simulink model "PSMPraga"  (R2021b)
settings: Solver=FixedStepDiscrete  StartTime=0.0  StopTime=8  RelTol=1e-3
PreLoadFcn:
  | Ts_Power=1e-6;
  | Ts_Control=100e-6;
undefined symbols (not defined in the file or in its folder): D1, Delta, DiscIntNeverNeededParam, sigbuilder_block
libraries: spsSeriesRLCBranchLib x10, spsVoltageMeasurementLib x10, slpidlib x8, spsPowerPositiveSequenceLib x8, spsCurrentMeasurementLib x8, spsThreePhaseVIMeasurementLib x6, eePowerMeasurement x6, spsabctodq0Lib x4, spsMeanLib x3, spsThreePhaseTransformerTwoWindingsLib x3, spsThreePhaseParallelRLCLoadLib x2, spsParallelRLCLoadLib x2
(part 1 of 3)
Description:
  | Copyright 2008-2019 The MathWorks, Inc.
settings Model: SimulationMode=accelerator  Creator=MathWorks  LastModifiedBy=user
settings SolverCC: AlgebraicLoopSolver=TrustRegion
settings DataIOCC: LimitDataPoints=on  SaveFormat=Array  SignalLoggingSaveFormat=ModelDataLogs  SignalLogging=off  DSMLogging=off  ReturnWorkspaceOutputs=off
settings OptimizationCC: ExpressionDepthLimit=2147483647  LifeSpan=inf
settings DebuggingCC: UnderspecifiedInitializationDetection=Classic  MergeDetectMultiDrivingBlocksExec=none  SolverPrmCheckMsg=warning  FcnCallInpInsideContextMsg=warning  StateNameClashWarn=warning  SFUnexpectedBacktrackingDiag=warning  SFNoUnconditionalDefaultTransitionDiag=warning  SFExecutionAtInitializationDiag=none  SFMachineParentedDataDiag=warning  ArithmeticOperatorsInVariantConditions=warning
settings HardwareCC: ProdBitPerPointer=32  ProdBitPerSizeT=32  ProdBitPerPtrDiffT=32  ProdLargestAtomicFloat=None  ProdIntDivRoundTo=Undefined  ProdEndianess=Unspecified  ProdWordSize=32  ProdHWDeviceType=32-bit Generic
settings ModelReferenceCC: PropagateSignalLabelsOutOfModel=off
settings SFSimCC: SimUseLocalCustomCode=off  CustomCodeUndefinedFunction=UseInterfaceOnly
settings RTWCC: RTWUseLocalCustomCode=off
settings CodeAppCC: StateflowObjectComments=on
settings GRTTargetCC: TargetLangStandard=C89/C90 (ANSI)  CombineOutputUpdateFcns=off  GRTInterface=on
settings ConfigComp: CovMetricSettings=dw  CovSaveCumulativeToWorkspaceVar=on  CovSaveSingleToWorkspaceVar=on  CovExternalEMLEnable=off  CovSFcnEnable=off
settings SimscapeCC: SimscapeNormalizeSystem=off

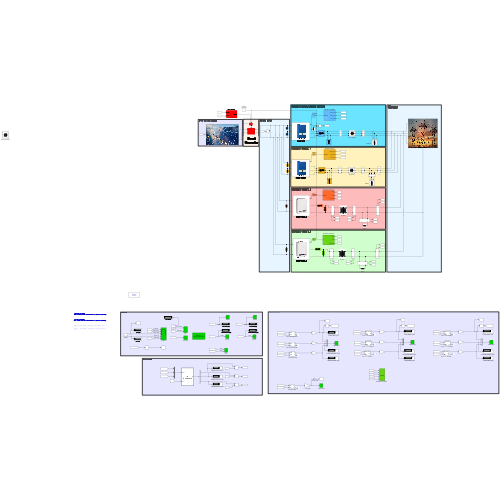
[thumbnail: Simulink's stored preview of the top-level diagram]
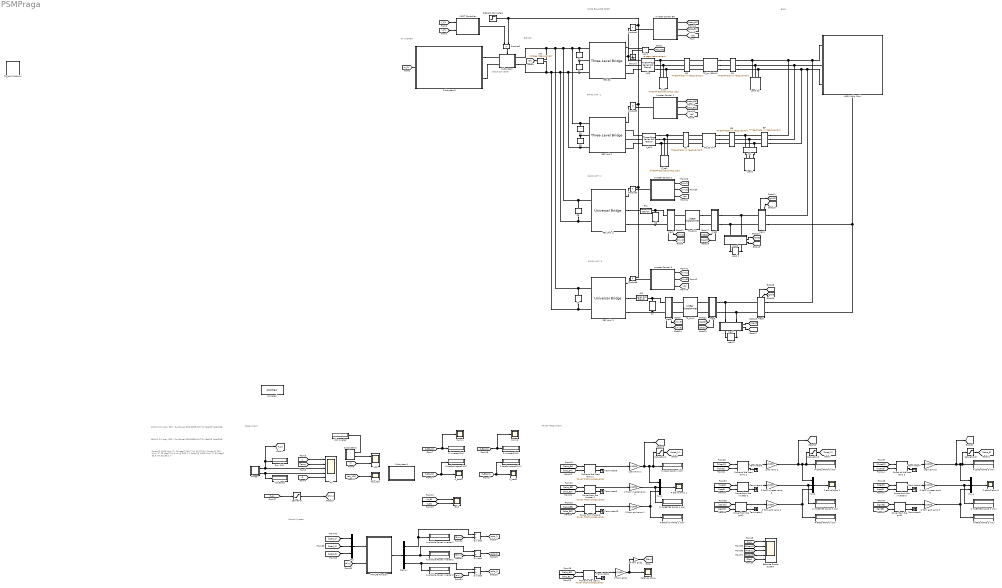
== system PSMPraga ==
  note: GRID
  note: RAMO UNIT. 3
  note: RAMO UNIT. 2
  note: RAMO UNIT. 1
  note: RAMO BALANCE NODE
  note: BUS DC
  note: PV SYSTEM
  note: Power Measurment
  note: Measurment
  note: Control System
  note: Boost Converter
  note: Pmpp @ 1000 W/m^2, 25 deg= 100.7 kW @ 273.5 V
      | Pmpp @  250 W/m^2, 25 deg= 24.4  kW @ 265.1 V
      | Pmpp @ 1000 W/m^2, 50 deg= 92.9  kW @ 250.2 V
  note: 100-kW  PV Array
      | 330 * SunPower SPR-305E-WHT-D  (Nser=5 Npar=66)
  note: 100-kW  PV Array
      | 330 * SunPower SPR-305E-WHT-D  (Nser=5 Npar=66)
  " Load SC" : spsThreePhaseParallelRLCLoadLib/Three-Phase Parallel RLC Load  LConnTagsString=A|B|C  Configuration=Y (grounded)  NominalVoltage=400  Vabc=[1e3 1e3 1e3]  Vabcp=[1e3 1e3 1e3]  NominalFrequency=50  UnbalancedPower=off  ActivePower=0.1  InductivePower=0  CapacitivePower=0  Pabc=[10e3 9e3 11e3]  QLabc=[100 90 110]  QCabc=[100 90 110]  Pabcp=[10e3 9e3 11e3]  QLabcp=[100 90 110]  QCabcp=[100 90 110]  Measurements=None  LoadType=constant Z
  " Load1" : spsThreePhaseParallelRLCLoadLib/Three-Phase Parallel RLC Load  LConnTagsString=A|B|C  Configuration=Y (grounded)  NominalVoltage=400  Vabc=[1e3 1e3 1e3]  Vabcp=[1e3 1e3 1e3]  NominalFrequency=50  UnbalancedPower=off  ActivePower=10000  InductivePower=0  CapacitivePower=0  Pabc=[10e3 9e3 11e3]  QLabc=[100 90 110]  QCabc=[100 90 110]  Pabcp=[10e3 9e3 11e3]  QLabcp=[100 90 110]  QCabcp=[100 90 110]  Measurements=None  LoadType=constant Z
  " Load 3" : spsParallelRLCLoadLib/Parallel RLC Load  LConnTagsString=a  RConnTagsString=__new0  NominalVoltage=230  NominalFrequency=50  ActivePower=3000  InductivePower=0  CapacitivePower=0  Setx0=off  InitialVoltage=0  SetiL0=off  InitialCurrent=0  Measurements=None  LoadType=constant Z
      settings: AttributesFormatString=\n  SourceProductBaseCode=PS
  600V Utlity Grid : Subsystem
      settings: PortSchema="{\"entries\":[{\"content\":{\"sides\":[{\"content\":{\"connectorIds\":[\"LConn1\",\"LConn2\",\"LConn3\"]},\"type\":\"ConnectorPlacement.EquallySpacedRectSide\",\"uuid\":\"36023811-46b7-429e-a8ab-d56566142e79\"},{\"content\":{\"connectorIds\":[],\"side\":\"RIGHT\"},\"type\":\"ConnectorPlacement.EquallySpacedRectSide\",\"uuid\":\"9af551aa-fa19-4e35-bdf3-eccb9cb0d58d\"},{\"content\":{\"connectorIds\":[],\"side\":\"TOP\"},\"type\":\"ConnectorPlacement.EquallySpacedRectSide\",\"uuid\":\"a2a5be34-f490-4bba-9aee-93a63d2f5fd5\"},{\"content\":{\"connectorIds\":[\"RConn1\"],\"side\":\"BOTTOM\"},\"type\":\"ConnectorPlacement.EquallySpacedRectSide\",\"uuid\":\"ebfc3acd-3bb4-47e0-af2a-a9fa1738ee4a\"}]},\"type\":\"ConnectorPlacement.EquallySpacedConnector\",\"uuid\":\"d54a4b0f-3adc-4ffb-80dc-ac1d592a2d32\"}],\"packageUris\":[\"http://schema.mathworks.com/mf0/Connector/R2020b\"],\"version\":\"1.0\"}"
      mask Display: image('$imagefile'); % Use "Edit Image" on toolstrip to change.
  Available Power Inverter 1 : Display
  Available Power Inverter 2 : Display
  Available Power Inverter 3 : Display
  B0 : spsThreePhaseVIMeasurementLib/Three-Phase V-I Measurement  VoltageMeasurement=phase-to-ground  SetLabelV=on  LabelV=Vabc_B0  Vpu=off  VpuLL=off  CurrentMeasurement=yes  SetLabelI=on  LabelI=Iabc_B0  Ipu=off  Pbase=100e6  Vbase=500e3  OutputType=Magnitude  PhasorSimulation=off  PSBequivalent=0
  B1 : spsThreePhaseVIMeasurementLib/Three-Phase V-I Measurement  VoltageMeasurement=phase-to-ground  SetLabelV=on  LabelV=Vabc_B1  Vpu=off  VpuLL=off  CurrentMeasurement=yes  SetLabelI=on  LabelI=Iabc_B1  Ipu=off  Pbase=100e6  Vbase=500e3  OutputType=Magnitude  PhasorSimulation=off  PSBequivalent=0
  B2 : spsThreePhaseVIMeasurementLib/Three-Phase V-I Measurement  VoltageMeasurement=phase-to-ground  SetLabelV=on  LabelV=Vabc_B2  Vpu=off  VpuLL=off  CurrentMeasurement=yes  SetLabelI=on  LabelI=Iabc_B2  Ipu=off  Pbase=100e6  Vbase=500e3  OutputType=Magnitude  PhasorSimulation=off  PSBequivalent=0
  B3 : spsThreePhaseVIMeasurementLib/Three-Phase V-I Measurement  VoltageMeasurement=phase-to-ground  SetLabelV=on  LabelV=Vabc_B3  Vpu=off  VpuLL=off  CurrentMeasurement=yes  SetLabelI=on  LabelI=Iabc_B3  Ipu=off  Pbase=100e6  Vbase=500e3  OutputType=Magnitude  PhasorSimulation=off  PSBequivalent=0
  B4 : spsThreePhaseVIMeasurementLib/Three-Phase V-I Measurement  VoltageMeasurement=phase-to-ground  SetLabelV=on  LabelV=Vabc_B4  Vpu=off  VpuLL=off  CurrentMeasurement=yes  SetLabelI=on  LabelI=Iabc_B4  Ipu=off  Pbase=100e6  Vbase=500e3  OutputType=Magnitude  PhasorSimulation=off  PSBequivalent=0
  B5 : spsThreePhaseVIMeasurementLib/Three-Phase V-I Measurement  VoltageMeasurement=phase-to-ground  SetLabelV=on  LabelV=Vabc_B5  Vpu=off  VpuLL=off  CurrentMeasurement=yes  SetLabelI=on  LabelI=Iabc_B5  Ipu=off  Pbase=100e6  Vbase=500e3  OutputType=Magnitude  PhasorSimulation=off  PSBequivalent=0
  Balance Power System : Scope  NumInputPorts=5
  C1 : spsSeriesRLCBranchLib/Series RLC Branch  LConnTagsString=__new0  RConnTagsString=__new0  BranchType=C  Resistance=1.0  Inductance=1.0  SetiL0=off  InitialCurrent=0  Capacitance=12000e-06  Setx0=off  InitialVoltage=0  Measurements=None
  C2 : spsSeriesRLCBranchLib/Series RLC Branch  LConnTagsString=__new0  RConnTagsString=__new0  BranchType=C  Resistance=1.0  Inductance=1.0  SetiL0=off  InitialCurrent=0  Capacitance=12000e-06  Setx0=off  InitialVoltage=0  Measurements=None
  C4 : spsSeriesRLCBranchLib/Series RLC Branch  LConnTagsString=__new0  RConnTagsString=__new0  BranchType=C  Resistance=1.0  Inductance=1.0  SetiL0=off  InitialCurrent=0  Capacitance=3000e-06  Setx0=off  InitialVoltage=0  Measurements=None
  C5 : spsSeriesRLCBranchLib/Series RLC Branch  LConnTagsString=__new0  RConnTagsString=__new0  BranchType=C  Resistance=1.0  Inductance=1.0  SetiL0=off  InitialCurrent=0  Capacitance=3000e-06  Setx0=off  InitialVoltage=0  Measurements=None
  C6 : spsSeriesRLCLoadLib/Series RLC Load  LConnTagsString=a  RConnTagsString=__new0  NominalVoltage=240  NominalFrequency=50  ActivePower=10e3/100  InductivePower=0  CapacitivePower=10e3  Setx0=off  InitialVoltage=0  SetiL0=off  InitialCurrent=0  Measurements=None  LoadType=constant Z
  C7 : spsSeriesRLCLoadLib/Series RLC Load  LConnTagsString=a  RConnTagsString=__new0  NominalVoltage=260  NominalFrequency=50  ActivePower=10e3/100  InductivePower=0  CapacitivePower=10e3  Setx0=off  InitialVoltage=0  SetiL0=off  InitialCurrent=0  Measurements=None  LoadType=constant Z
  C8 : spsSeriesRLCBranchLib/Series RLC Branch  LConnTagsString=__new0  RConnTagsString=__new0  BranchType=C  Resistance=1.0  Inductance=1.0  SetiL0=off  InitialCurrent=0  Capacitance=9000e-06  Setx0=off  InitialVoltage=0  Measurements=None
  C9 : spsSeriesRLCBranchLib/Series RLC Branch  LConnTagsString=__new0  RConnTagsString=__new0  BranchType=C  Resistance=1.0  Inductance=1.0  SetiL0=off  InitialCurrent=0  Capacitance=10000e-06  Setx0=off  InitialVoltage=0  Measurements=None
  C_ba : spsThreePhaseSeriesRLCLoadLib/Three-Phase Series RLC Load  LConnTagsString=A|B|C  Configuration=Y (grounded)  NominalVoltage=260  Vabc=[1e3 1e3 1e3]  Vabcp=[1e3 1e3 1e3]  NominalFrequency=50  UnbalancedPower=off  ActivePower=10e3/100  InductivePower=0  CapacitivePower=10e3  Pabc=[10e3 9e3 11e3]  QLabc=[100 90 110]  QCabc=[100 90 110]  Pabcp=[10e3 9e3 11e3]  QLabcp=[100 90 110]  QCabcp=[100 90 110]  Measurements=None  LoadType=constant Z
  C_ba1 : spsThreePhaseSeriesRLCLoadLib/Three-Phase Series RLC Load  LConnTagsString=A|B|C  Configuration=Y (grounded)  NominalVoltage=260  Vabc=[1e3 1e3 1e3]  Vabcp=[1e3 1e3 1e3]  NominalFrequency=50  UnbalancedPower=off  ActivePower=10e3/100  InductivePower=0  CapacitivePower=10e3  Pabc=[10e3 9e3 11e3]  QLabc=[100 90 110]  QCabc=[100 90 110]  Pabcp=[10e3 9e3 11e3]  QLabcp=[100 90 110]  QCabcp=[100 90 110]  Measurements=None  LoadType=constant Z
  Deblock Converters : Step  Time=0.05  SampleTime=0
  Demux : Demux  Outputs=3
  Divide3 : Product  Inputs=*/
  Divide4 : Product  Inputs=*/
  Divide5 : Product  Inputs=*/
  FEC BN : spsThreeLevelBridgeLib/Three-Level Bridge  Arms=3  SnubberResistance=1e6  SbubberCapacitance=inf  Device=IGBT / Diodes  Ron=0.2e-3  ForwardVoltages="[  0  0 ]"  Measurements=None  mask(Three-Level Bridge){}
      settings: AttributesFormatString=\n  SourceProductBaseCode=PS
      mask Display: image('C:\Users\user\Desktop\Matlab\Immagini\inverter trifase.jpg'); % Use "Edit Image" on toolstrip to change.
  FEC Unit. 2 : spsUniversalBridgeLib/Universal Bridge  Arms=2  SnubberResistance=1e6  SnubberCapacitance=inf  Device=IGBT / Diodes  Ron=0.2e-3  Lon=0  ForwardVoltages="[  0  0  ]"  ForwardVoltage=0  GTOparameters=[ 10e-6 , 20e-6 ]  IGBTparameters=[ 1e-6 , 2e-6 ]  Measurements=None  Measurements_2=None  converterType=Rectifier  mask(Universal Bridge){}
      mask Display: image('C:\Users\user\Desktop\Matlab\Immagini\inveter monofase.jpg'); % Use "Edit Image" on toolstrip to change.
  FEC Unit. 3 : spsUniversalBridgeLib/Universal Bridge  Arms=2  SnubberResistance=1e6  SnubberCapacitance=inf  Device=IGBT / Diodes  Ron=0.2e-3  Lon=0  ForwardVoltages="[  0  0  ]"  ForwardVoltage=0  GTOparameters=[ 10e-6 , 20e-6 ]  IGBTparameters=[ 1e-6 , 2e-6 ]  Measurements=None  Measurements_2=None  converterType=Rectifier  mask(Universal Bridge){}
      mask Display: image('C:\Users\user\Desktop\Matlab\Immagini\inveter monofase.jpg'); % Use "Edit Image" on toolstrip to change.
  FEC Unit.1 : spsThreeLevelBridgeLib/Three-Level Bridge  Arms=3  SnubberResistance=1e6  SbubberCapacitance=inf  Device=IGBT / Diodes  Ron=0.2e-3  ForwardVoltages="[0  0 ]"  Measurements=None  mask(Three-Level Bridge){}
      settings: AttributesFormatString=\n  SourceProductBaseCode=PS
      mask Display: image('C:\Users\user\Desktop\Matlab\Immagini\inverter trifase.jpg'); % Use "Edit Image" on toolstrip to change.
  Grid : Scope  NumInputPorts=2
  Ground : spsGroundLib/Ground  LConnTagsString=a
  Inverter Control 1 : Subsystem  mask(VSC Main Controller){nom=[10e3  50 ], Vnom=[400 260 ], Vnom_dc=500, RLxfo=[0.002  0.06], RLchoke=[0.0075 250e-6], K_VDCreg=[7 800], K_Ireg=[0.3 20], Ts=Ts_Control}
      mask prompts: nom "Nominal power and frequency [ Pnom(VA)  Fnom(Hz) ]:"; Vnom "Nominal primary and secondary voltages (Vrms LL) [ Vnom_prim   Vnom_sec ]:"; Vnom_dc "Nominal DC bus voltage (V):"; RLxfo "Total transformer leakage impedance (pu/Pnom) [ Rxfo  Lxf ]"; RLchoke "Choke impedance [ R(ohm) L(H) ]"; K_VDCreg "VDC regultator gains [ Kp  Ki ]:"; K_Ireg "Current regulator gains [ Kp  Ki ]:"; Ts "Sample time"
      mask init:
      | Pnom=nom(1);
      | Fnom=nom(2);
      | Vnom_prim=Vnom(1);
      | Vnom_sec=Vnom(2);
      | Zbase=(Vnom_sec^2/(Pnom*10));
      | Rtot_pu=RLxfo(1) + RLchoke(1)/Zbase;
      | Ltot_pu=RLxfo(2) + RLchoke(2)/(Zbase/(2*pi*Fnom));
      | Kp_VDCreg=K_VDCreg(1);
      | Ki_VDCreg=K_VDCreg(2);
      | Kp_Ireg=K_Ireg(1);
      | Ki_Ireg=K_Ireg(2);
      | Vdc_ref=Vnom_dc;
      | % Used to determine initial value of Boost Control (MPPT)
      | assignin('base','Vdc_ref_Inv',Vdc_ref);
  Inverter Control 2 : Subsystem  mask(Inverter Control){Pnom=6000, Fnom=50, Vnom_sec=260, Vnom_dc=500, Kp_VDCreg=7, Ki_VDCreg=800, Kp_Ireg=0.30, Ki_Ireg=20, RLxfo=[0.002  0.06], RLchoke=[2e-3  1.78e-3], Fc=1650, PWMmode12=Bipolar, Ts_Control=Ts_Control, Ts_PWMgenerator=Ts_Power}
      mask prompts: Pnom "Nominal Power (VA)"; Fnom "Frequency (Hz)"; Vnom_sec "Secondary voltage (Vrms LN)"; Vnom_dc "DC BUS voltage nominal (V)"; Kp_VDCreg "Proportional gain"; Ki_VDCreg "Integral gain"; Kp_Ireg "Proportional gain"; Ki_Ireg "Integral gain"; RLxfo "Total transformer leakage impedance (pu/Pnom) [ Rxfo  Lxf ]"; RLchoke "Choke impedance [ R(ohm) L(H) ]"; Fc "Carrier frequency (Hz)"; PWMmode12 "PWM method"; Ts_Control "Control systems"; Ts_PWMgenerator "PWM generator"
      mask help:
      | The main components of the Inverter Control are:
      | 1. PLL & Measurements
      | 2. Maximum Power Point Tracker System (MPPT) using a Perturb & Observe algorithm
      | 3. DC Voltage Regulator
      | 4. Current Regulator
      | 5. PWM Modulator
      mask init:
      | blockName=gcb;
      | Vdc_ref=Vnom_dc;
      | Zbase=Vnom_sec^2/(Pnom*3);
      | Rtot_pu=RLxfo(1) + RLchoke(1)/Zbase;
      | Ltot_pu=RLxfo(2) + RLchoke(2)/(Zbase/(2*pi*Fnom));
      | if PWMmode12==1
      |     set_param([blockName,'/','PWM_Generator'],'ModulatorType','Single-phase full-bridge (4 pulses)')
      | else
      |     set_param([blockName,'/','PWM_Generator'],'ModulatorType','Single-phase full-bridge - Bipolar modulation (4 pulses)')
      | end
      mask TypeOptions PWMmode12: Unipolar | Bipolar
      mask DialogControl Container4 Prompt: Nominal Values:
      mask DialogControl Container8 Prompt: Dc Voltage Regulator:
      mask DialogControl Container6 Prompt: Current Regulator:
      mask DialogControl Container9 Prompt: PWM Modulator:
      mask DialogControl SampleTimes Prompt: Sample Times:
  Inverter Control 3 : Subsystem  mask(Inverter Control){Pnom=3000, Fnom=50, Vnom_sec=260, Vnom_dc=500, Kp_VDCreg=7, Ki_VDCreg=800, Kp_Ireg=0.30, Ki_Ireg=20, RLxfo=[0.0002  0.000019], RLchoke=[2e-3  1.78e-3], Fc=1650, PWMmode12=Bipolar, Ts_Control=Ts_Control, Ts_PWMgenerator=Ts_Power}
      mask prompts: Pnom "Nominal Power (VA)"; Fnom "Frequency (Hz)"; Vnom_sec "Secondary voltage (Vrms LN)"; Vnom_dc "DC BUS voltage nominal (V)"; Kp_VDCreg "Proportional gain"; Ki_VDCreg "Integral gain"; Kp_Ireg "Proportional gain"; Ki_Ireg "Integral gain"; RLxfo "Total transformer leakage impedance (pu/Pnom) [ Rxfo  Lxf ]"; RLchoke "Choke impedance [ R(ohm) L(H) ]"; Fc "Carrier frequency (Hz)"; PWMmode12 "PWM method"; Ts_Control "Control systems"; Ts_PWMgenerator "PWM generator"
      mask help:
      | The main components of the Inverter Control are:
      | 1. PLL & Measurements
      | 2. Maximum Power Point Tracker System (MPPT) using a Perturb & Observe algorithm
      | 3. DC Voltage Regulator
      | 4. Current Regulator
      | 5. PWM Modulator
      mask init:
      | blockName=gcb;
      | Vdc_ref=Vnom_dc;
      | Zbase=Vnom_sec^2/Pnom;
      | Rtot_pu=RLxfo(1) + RLchoke(1)/Zbase;
      | Ltot_pu=RLxfo(2) + RLchoke(2)/(Zbase/(2*pi*Fnom));
      | if PWMmode12==1
      |     set_param([blockName,'/','PWM_Generator'],'ModulatorType','Single-phase full-bridge (4 pulses)')
      | else
      |     set_param([blockName,'/','PWM_Generator'],'ModulatorType','Single-phase full-bridge - Bipolar modulation (4 pulses)')
      | end
      mask TypeOptions PWMmode12: Unipolar | Bipolar
      mask DialogControl Container4 Prompt: Nominal Values:
      mask DialogControl Container8 Prompt: Dc Voltage Regulator:
      mask DialogControl Container6 Prompt: Current Regulator:
      mask DialogControl Container9 Prompt: PWM Modulator:
      mask DialogControl SampleTimes Prompt: Sample Times:
  Inverter Control BN : Subsystem  mask(VSC Main Controller){nom=[30e3  50 ], Vnom=[ 400 260 ], Vnom_dc=500, RLxfo=[0.002  0.06 ], RLchoke=[2e-3  250e-6  ], K_VDCreg=[7  800], K_Ireg=[0.3 20], Ts=Ts_Control}
      mask prompts: nom "Nominal power and frequency [ Pnom(VA)  Fnom(Hz) ]:"; Vnom "Nominal primary and secondary voltages (Vrms LL) [ Vnom_prim   Vnom_sec ]:"; Vnom_dc "Nominal DC bus voltage (V):"; RLxfo "Total transformer leakage impedance (pu/Pnom) [ Rxfo  Lxf ]"; RLchoke "Choke impedance [ R(ohm) L(H) ]"; K_VDCreg "VDC regultator gains [ Kp  Ki ]:"; K_Ireg "Current regulator gains [ Kp  Ki ]:"; Ts "Sample time"
      mask init:
      | Pnom=nom(1);
      | Fnom=nom(2);
      | Vnom_prim=Vnom(1);
      | Vnom_sec=Vnom(2);
      | Zbase=Vnom_sec^2/(Pnom*10/3);
      | Rtot_pu=RLxfo(1) + RLchoke(1)/Zbase;
      | Ltot_pu=RLxfo(2) + RLchoke(2)/(Zbase/(2*pi*Fnom));
      | Kp_VDCreg=K_VDCreg(1);
      | Ki_VDCreg=K_VDCreg(2);
      | Kp_Ireg=K_Ireg(1);
      | Ki_Ireg=K_Ireg(2);
      | Vdc_ref=Vnom_dc;
      | % Used to determine initial value of Boost Control (MPPT)
      | assignin('base','Vdc_ref_Inv',Vdc_ref);
  L_ba : spsThreePhaseSeriesRLCBranchLib/Three-Phase Series RLC Branch  LConnTagsString=A|B|C  RConnTagsString=A|B|C  BranchType=RL  Resistance=500e-6*377/50/2  Inductance=500e-6/2  Capacitance=inf  Measurements=None
  L_ba1 : spsThreePhaseSeriesRLCBranchLib/Three-Phase Series RLC Branch  LConnTagsString=A|B|C  RConnTagsString=A|B|C  BranchType=RL  Resistance=500e-6*377/50/2  Inductance=250e-6  Capacitance=inf  Measurements=None
  Load 2 : spsParallelRLCLoadLib/Parallel RLC Load  LConnTagsString=a  RConnTagsString=__new0  NominalVoltage=230  NominalFrequency=50  ActivePower=6000  InductivePower=0  CapacitivePower=0  Setx0=off  InitialVoltage=0  SetiL0=off  InitialCurrent=0  Measurements=None  LoadType=constant Z
      settings: AttributesFormatString=\n  SourceProductBaseCode=PS
  "Load ramo 1 " : Gain  Gain=1/1000
  Load ramo 2 : Gain  Gain=1/1000
  Load ramo 3 : Gain  Gain=1/1000
  MATLAB Function : MATLAB Function  TreatAsAtomicUnit=on
  MPPT Controller : Subsystem  mask(Boost Control - MPPT){fc=5000, T_MPPT=200e-6, Dinit=0.5}
      mask prompts: fc "PWM switching frequency (Hz)"; T_MPPT "Time window used by MPPT control (s)"; Dinit "Initial value of duty cycle"
  Mux{,1,3..4} (4 alike) : Mux  Inputs=3
  P GRID RAMO 2 (kW) : Display
      settings: Format=bank
  P GRID RAMO 3 (kW) : Display
      settings: Format=bank
  P GRID kW RAMO 1 (kW) : Display
  P INVERTER RAMO 1 (kW) : Display
  P INVERTER RAMO 2 (kW) : Display
      settings: Format=bank
  P INVERTER RAMO 3 (kW) : Display
      settings: Format=bank
  P LOAD RAMO 1 (kW) : Display
  P LOAD RAMO 2 (kW) : Display
      settings: Format=bank
  P LOAD RAMO 3 (kW) : Display
      settings: Format=bank
  P attiva ramo 1 : Scope
  P attiva ramo 2 : Scope
  P attiva ramo 3 : Scope
  P from grid ramo 1 : Gain  Gain=1/1000
  P from grid ramo 2 : Gain  Gain=1/1000
  P from grid ramo 3 : Gain  Gain=1/1000
  P from grid1 : Gain  Gain=1/1000
  P from grid2 : Gain  Gain=-1
  P from inverter ramo 1 : Gain  Gain=1/1000
  P from inverter ramo 2 : Gain  Gain=1/1000
  P from inverter ramo 3 : Gain  Gain=1/1000
  P inverter1(kW) : Display
      settings: Format=bank  Decimation=2000
  P inverter2(kW) : Display
      settings: Format=bank  Decimation=2000
  P trasformatore1(kW) : Display
      settings: Format=bank  Decimation=2000
  P trasformatore2(kW) : Display
      settings: Format=bank  Decimation=2000
  PV : Scope  NumInputPorts=5
  P_Inv1 : Scope
  P_Inv2 : Scope
  P_trasf1 : Scope
  P_trasf2 : Scope
  Pmean : Subsystem
  Potenza Attiva : Scope
  Power from the grid : spsPowerPositiveSequenceLib/Power (Positive-Sequence)  Freq=50  Vinit=[0, 0]  Iinit=[0, 0]  Ts=Ts_Control
      settings: SourceProductBaseCode=PS
  Power from the grid1 : eePowerMeasurement/Power Measurement  LabelModeActiveChoice=Discrete  F=50  K=[1]  Ts=Ts_Control
      settings: SourceProductBaseCode=PS
  Power from the grid2 : eePowerMeasurement/Power Measurement  LabelModeActiveChoice=Discrete  F=50  K=[1]  Ts=Ts_Control
      settings: SourceProductBaseCode=PS
  Power from the inverter 1 : spsPowerPositiveSequenceLib/Power (Positive-Sequence)  Freq=50  Vinit=[0, 0]  Iinit=[0, 0]  Ts=Ts_Control
      settings: SourceProductBaseCode=PS
  Power from the inverter 2 : eePowerMeasurement/Power Measurement  LabelModeActiveChoice=Discrete  F=50  K=[1]  Ts=Ts_Control
      settings: SourceProductBaseCode=PS
  Power from the inverter 3 : eePowerMeasurement/Power Measurement  LabelModeActiveChoice=Discrete  F=50  K=[1]  Ts=Ts_Control
      settings: SourceProductBaseCode=PS
  Power to the load 1 : spsPowerPositiveSequenceLib/Power (Positive-Sequence)  Freq=50  Vinit=[0, 0]  Iinit=[0, 0]  Ts=Ts_Control
      settings: SourceProductBaseCode=PS
  "Power to the load ramo 1 " : spsPowerPositiveSequenceLib/Power (Positive-Sequence)  Freq=50  Vinit=[0, 0]  Iinit=[0, 0]  Ts=Ts_Control
      settings: SourceProductBaseCode=PS
  Power to the load ramo 2 : eePowerMeasurement/Power Measurement  LabelModeActiveChoice=Discrete  F=50  K=[1]  Ts=Ts_Control
      settings: SourceProductBaseCode=PS
  Power to the load ramo 3 : eePowerMeasurement/Power Measurement  LabelModeActiveChoice=Discrete  F=50  K=[1]  Ts=Ts_Control
      settings: SourceProductBaseCode=PS
  "Ppv (kW) " : Display
      settings: Format=bank  Decimation=2000
  Product{1..5} (5 alike) : Product  RndMeth=Zero
  RL1 : spsSeriesRLCBranchLib/Series RLC Branch  LConnTagsString=__new0  RConnTagsString=__new0  BranchType=RL  Resistance=1.78e-3  Inductance=1.78e-3  SetiL0=off  InitialCurrent=0  Capacitance=1e-6  Setx0=off  InitialVoltage=0  Measurements=None
  RL2 : spsSeriesRLCBranchLib/Series RLC Branch  LConnTagsString=__new0  RConnTagsString=__new0  BranchType=RL  Resistance=2e-3  Inductance=1.78e-3  SetiL0=off  InitialCurrent=0  Capacitance=1e-6  Setx0=off  InitialVoltage=0  Measurements=None
  Saturation : Saturate  UpperLimit=inf  LowerLimit=5
  Saturation1 : Saturate  UpperLimit=10  LowerLimit=0
  Saturation2 : Saturate  UpperLimit=6  LowerLimit=0
  Saturation3 : Saturate  UpperLimit=3  LowerLimit=0
  Subsystem : Subsystem
      settings: PortSchema="{\"entries\":[{\"content\":{\"sides\":[{\"content\":{\"connectorIds\":[\"LConn1\",\"LConn2\"]},\"type\":\"ConnectorPlacement.EquallySpacedRectSide\",\"uuid\":\"3e835128-e9bc-4b38-99ef-503abca9e331\"},{\"content\":{\"connectorIds\":[\"RConn1\",\"RConn2\"],\"side\":\"RIGHT\"},\"type\":\"ConnectorPlacement.EquallySpacedRectSide\",\"uuid\":\"e2d512d1-2b93-42a3-a0d9-5f9788cc5947\"},{\"content\":{\"connectorIds\":[\"In1\"],\"side\":\"TOP\"},\"type\":\"ConnectorPlacement.EquallySpacedRectSide\",\"uuid\":\"d62533dd-12de-41ca-a762-f41dfda2dc51\"}]},\"type\":\"ConnectorPlacement.EquallySpacedConnector\",\"uuid\":\"56877a3f-7e23-4e4a-9396-bd4c14571757\"}],\"packageUris\":[\"http://schema.mathworks.com/mf0/Connector/R2020b\"],\"version\":\"1.0\"}"
  Subsystem1 : Subsystem
      mask Display: disp('additional \nscopes & measurements')
  Subsystem2 : Subsystem
  Subsystem3 : Subsystem
      settings: PortSchema="{\"entries\":[{\"content\":{\"sides\":[{\"content\":{\"connectorIds\":[\"Out1\"]},\"type\":\"ConnectorPlacement.EquallySpacedRectSide\",\"uuid\":\"68e7d602-4857-4e8c-a67c-1310801dcc61\"},{\"content\":{\"connectorIds\":[\"RConn1\",\"RConn2\"],\"side\":\"RIGHT\"},\"type\":\"ConnectorPlacement.EquallySpacedRectSide\",\"uuid\":\"62fc7201-c46d-4754-9ff1-5573421867bb\"},{\"content\":{\"connectorIds\":[],\"side\":\"TOP\"},\"type\":\"ConnectorPlacement.EquallySpacedRectSide\",\"uuid\":\"c27e8248-44f7-4229-afdb-9dd416acee4c\"}]},\"type\":\"ConnectorPlacement.EquallySpacedConnector\",\"uuid\":\"379c0bbc-daf5-42fe-b22b-bdfe688145b7\"}],\"packageUris\":[\"http://schema.mathworks.com/mf0/Connector/R2020b\"],\"version\":\"1.0\"}"
      mask Display: image('C:\Users\user\Desktop\Matlab\Immagini\14.11-Moduli-FV-bifacciali-936x527.jpg'); % Use "Edit Image" on toolstrip to change.
  "TR_10 kVA " : spsThreePhaseTransformerTwoWindingsLib/Three-Phase Transformer (Two Windings)  Winding1Connection=Yg  Winding2Connection=Delta (D1)  CoreType=Three single-phase transformers  SetSaturation=off  Hysteresis=off  DataFile='hysteresis'  SetInitialFlux=off  Measurements=None  UNITS=pu  NominalPower=[ 10e3 , 50 ]  Winding1=[400 0.001 0.03]  Winding2=[260 0.001 0.03]  Rm=500  Lm=500  L0=0.5  Saturation=[0 0;0.0024 1.2;0.99998 1.52]  InitialFluxes=[-1.03972409712903 0.521706895887502 0.518017201241549]  BreakLoop=off  DiscreteSolver=Trapezoidal iterative  DataType=off  TransfoNumber=0
  TR_3kVA : spsLinearTransformerLib/Linear Transformer  UNITS=SI  NominalPower=[ 3e3 50 ]  winding1=[230 0.0017633 0.00016839]  winding2=[260 0.0022533 0.00021518]  ThreeWindings=off  winding3=[115 0.0044083 0.00042096]  RmLm=[17633 56.129]  Measurements=None  DataType=on
  TR_6kVA : spsLinearTransformerLib/Linear Transformer  UNITS=pu  NominalPower=[ 6e3 50 ]  winding1=[230 0.0001 0.0030001]  winding2=[260 0.0001 0.003]  ThreeWindings=off  winding3=[115 0.00099997 0.03]  RmLm=[500 499.99]  Measurements=None  DataType=off
  TR_bn (30kVA) : spsThreePhaseTransformerTwoWindingsLib/Three-Phase Transformer (Two Windings)  Winding1Connection=Yg  Winding2Connection=Delta (D1)  CoreType=Three single-phase transformers  SetSaturation=off  Hysteresis=off  DataFile='hysteresis'  SetInitialFlux=off  Measurements=None  UNITS=pu  NominalPower=[30e3 , 50 ]  Winding1=[400 0.00099999 0.003]  Winding2=[260 0.001 0.003]  Rm=500  Lm=500  L0=1734.9  Saturation=[0 0;0.008 1.2;3.3333 1.52]  InitialFluxes=[0.74022 -0.74022 0.64769]  BreakLoop=off  DiscreteSolver=Trapezoidal iterative  DataType=off  TransfoNumber=0
  TR_bn1 (100kVA) : spsThreePhaseTransformerTwoWindingsLib/Three-Phase Transformer (Two Windings)  Winding1Connection=Yg  Winding2Connection=Delta (D1)  CoreType=Three single-phase transformers  SetSaturation=off  Hysteresis=off  DataFile='hysteresis'  SetInitialFlux=off  Measurements=None  UNITS=pu  NominalPower=[100e3 , 50 ]  Winding1=[400 0.001 0.03]  Winding2=[260 0.001 0.03]  Rm=500  Lm=500  L0=0.5  Saturation=[0 0;0.0024 1.2;0.99998 1.52]  InitialFluxes=[0.8 -0.8 0.7]  BreakLoop=off  DiscreteSolver=Trapezoidal iterative  DataType=off  TransfoNumber=0
  Terminator{1..10} (10 alike) : Terminator
  VSC : Scope  NumInputPorts=2
  Vab_VSC : Scope
  "Vdc " : spsVoltageMeasurementLib/Voltage Measurement  Tag=PoWeRsYsTeMmEaSuReMeNt  PhasorSimulation=off  OutputType=Magnitude  PSBequivalent=0
  Vdc 1 : spsVoltageMeasurementLib/Voltage Measurement  Tag=PoWeRsYsTeMmEaSuReMeNt  PhasorSimulation=off  OutputType=Magnitude  PSBequivalent=0
  Vdc Boost : Display
      settings: Format=bank  Decimation=2000
  Vdc Inverter : Display
      settings: Format=bank  Decimation=2000
  mes1 : Subsystem
      settings: PortSchema="{\"entries\":[{\"content\":{\"sides\":[{\"content\":{\"connectorIds\":[\"LConn1\",\"LConn2\"]},\"type\":\"ConnectorPlacement.EquallySpacedRectSide\",\"uuid\":\"063d70f7-53e6-4b16-b677-e8cc0b373f72\"},{\"content\":{\"connectorIds\":[\"RConn1\",\"RConn2\"],\"side\":\"RIGHT\"},\"type\":\"ConnectorPlacement.EquallySpacedRectSide\",\"uuid\":\"e5801cd5-69d1-49e6-883b-eb22ff99f49e\"},{\"content\":{\"connectorIds\":[],\"side\":\"TOP\"},\"type\":\"ConnectorPlacement.EquallySpacedRectSide\",\"uuid\":\"e62b0121-10a9-4e1e-945c-5e32104486a2\"},{\"content\":{\"connectorIds\":[\"Out1\",\"Out2\"],\"side\":\"BOTTOM\"},\"type\":\"ConnectorPlacement.EquallySpacedRectSide\",\"uuid\":\"615cb022-86c8-4d65-b4a5-653fc637b1c5\"}]},\"type\":\"ConnectorPlacement.EquallySpacedConnector\",\"uuid\":\"b7a6c70d-1829-427f-bdc0-db8f4193df4b\"}],\"packageUris\":[\"http://schema.mathworks.com/mf0/Connector/R2020b\"],\"version\":\"1.0\"}"
  mes2 : Subsystem
      settings: PortSchema="{\"entries\":[{\"content\":{\"sides\":[{\"content\":{\"connectorIds\":[\"LConn1\",\"LConn2\"]},\"type\":\"ConnectorPlacement.EquallySpacedRectSide\",\"uuid\":\"063d70f7-53e6-4b16-b677-e8cc0b373f72\"},{\"content\":{\"connectorIds\":[\"RConn1\",\"RConn2\"],\"side\":\"RIGHT\"},\"type\":\"ConnectorPlacement.EquallySpacedRectSide\",\"uuid\":\"e5801cd5-69d1-49e6-883b-eb22ff99f49e\"},{\"content\":{\"connectorIds\":[],\"side\":\"TOP\"},\"type\":\"ConnectorPlacement.EquallySpacedRectSide\",\"uuid\":\"e62b0121-10a9-4e1e-945c-5e32104486a2\"},{\"content\":{\"connectorIds\":[\"Out1\",\"Out2\"],\"side\":\"BOTTOM\"},\"type\":\"ConnectorPlacement.EquallySpacedRectSide\",\"uuid\":\"13dcf0ef-fcc5-4001-9759-8913e91797b5\"}]},\"type\":\"ConnectorPlacement.EquallySpacedConnector\",\"uuid\":\"b7a6c70d-1829-427f-bdc0-db8f4193df4b\"}],\"packageUris\":[\"http://schema.mathworks.com/mf0/Connector/R2020b\"],\"version\":\"1.0\"}"
  mes3 : Subsystem
      settings: PortSchema="{\"entries\":[{\"content\":{\"sides\":[{\"content\":{\"connectorIds\":[\"LConn1\",\"LConn2\"]},\"type\":\"ConnectorPlacement.EquallySpacedRectSide\",\"uuid\":\"063d70f7-53e6-4b16-b677-e8cc0b373f72\"},{\"content\":{\"connectorIds\":[\"RConn1\",\"RConn2\"],\"side\":\"RIGHT\"},\"type\":\"ConnectorPlacement.EquallySpacedRectSide\",\"uuid\":\"e5801cd5-69d1-49e6-883b-eb22ff99f49e\"},{\"content\":{\"connectorIds\":[\"Out1\",\"Out2\"],\"side\":\"TOP\"},\"type\":\"ConnectorPlacement.EquallySpacedRectSide\",\"uuid\":\"e62b0121-10a9-4e1e-945c-5e32104486a2\"}]},\"type\":\"ConnectorPlacement.EquallySpacedConnector\",\"uuid\":\"b7a6c70d-1829-427f-bdc0-db8f4193df4b\"}],\"packageUris\":[\"http://schema.mathworks.com/mf0/Connector/R2020b\"],\"version\":\"1.0\"}"
  mes4 : Subsystem
      settings: PortSchema="{\"entries\":[{\"content\":{\"sides\":[{\"content\":{\"connectorIds\":[\"LConn1\",\"LConn2\"]},\"type\":\"ConnectorPlacement.EquallySpacedRectSide\",\"uuid\":\"063d70f7-53e6-4b16-b677-e8cc0b373f72\"},{\"content\":{\"connectorIds\":[\"RConn1\",\"RConn2\"],\"side\":\"RIGHT\"},\"type\":\"ConnectorPlacement.EquallySpacedRectSide\",\"uuid\":\"e5801cd5-69d1-49e6-883b-eb22ff99f49e\"},{\"content\":{\"connectorIds\":[\"Out1\",\"Out2\"],\"side\":\"TOP\"},\"type\":\"ConnectorPlacement.EquallySpacedRectSide\",\"uuid\":\"e62b0121-10a9-4e1e-945c-5e32104486a2\"}]},\"type\":\"ConnectorPlacement.EquallySpacedConnector\",\"uuid\":\"b7a6c70d-1829-427f-bdc0-db8f4193df4b\"}],\"packageUris\":[\"http://schema.mathworks.com/mf0/Connector/R2020b\"],\"version\":\"1.0\"}"
  mes5 : Subsystem
      settings: PortSchema="{\"entries\":[{\"content\":{\"sides\":[{\"content\":{\"connectorIds\":[\"LConn1\",\"LConn2\"]},\"type\":\"ConnectorPlacement.EquallySpacedRectSide\",\"uuid\":\"063d70f7-53e6-4b16-b677-e8cc0b373f72\"},{\"content\":{\"connectorIds\":[\"RConn1\",\"RConn2\"],\"side\":\"RIGHT\"},\"type\":\"ConnectorPlacement.EquallySpacedRectSide\",\"uuid\":\"e5801cd5-69d1-49e6-883b-eb22ff99f49e\"},{\"content\":{\"connectorIds\":[],\"side\":\"TOP\"},\"type\":\"ConnectorPlacement.EquallySpacedRectSide\",\"uuid\":\"e62b0121-10a9-4e1e-945c-5e32104486a2\"},{\"content\":{\"connectorIds\":[\"Out1\",\"Out2\"],\"side\":\"BOTTOM\"},\"type\":\"ConnectorPlacement.EquallySpacedRectSide\",\"uuid\":\"ad074cc7-7126-462e-a1e8-556088d141fb\"}]},\"type\":\"ConnectorPlacement.EquallySpacedConnector\",\"uuid\":\"b7a6c70d-1829-427f-bdc0-db8f4193df4b\"}],\"packageUris\":[\"http://schema.mathworks.com/mf0/Connector/R2020b\"],\"version\":\"1.0\"}"
  mes6 : Subsystem
      settings: PortSchema="{\"entries\":[{\"content\":{\"sides\":[{\"content\":{\"connectorIds\":[\"LConn1\",\"LConn2\"]},\"type\":\"ConnectorPlacement.EquallySpacedRectSide\",\"uuid\":\"063d70f7-53e6-4b16-b677-e8cc0b373f72\"},{\"content\":{\"connectorIds\":[\"RConn1\",\"RConn2\"],\"side\":\"RIGHT\"},\"type\":\"ConnectorPlacement.EquallySpacedRectSide\",\"uuid\":\"e5801cd5-69d1-49e6-883b-eb22ff99f49e\"},{\"content\":{\"connectorIds\":[],\"side\":\"TOP\"},\"type\":\"ConnectorPlacement.EquallySpacedRectSide\",\"uuid\":\"e62b0121-10a9-4e1e-945c-5e32104486a2\"},{\"content\":{\"connectorIds\":[\"Out1\",\"Out2\"],\"side\":\"BOTTOM\"},\"type\":\"ConnectorPlacement.EquallySpacedRectSide\",\"uuid\":\"58c3191b-fb4d-4c54-8fba-d55eebfb88aa\"}]},\"type\":\"ConnectorPlacement.EquallySpacedConnector\",\"uuid\":\"b7a6c70d-1829-427f-bdc0-db8f4193df4b\"}],\"packageUris\":[\"http://schema.mathworks.com/mf0/Connector/R2020b\"],\"version\":\"1.0\"}"
  mes7 : Subsystem
      settings: PortSchema="{\"entries\":[{\"content\":{\"sides\":[{\"content\":{\"connectorIds\":[\"LConn1\",\"LConn2\"]},\"type\":\"ConnectorPlacement.EquallySpacedRectSide\",\"uuid\":\"063d70f7-53e6-4b16-b677-e8cc0b373f72\"},{\"content\":{\"connectorIds\":[\"RConn1\",\"RConn2\"],\"side\":\"RIGHT\"},\"type\":\"ConnectorPlacement.EquallySpacedRectSide\",\"uuid\":\"e5801cd5-69d1-49e6-883b-eb22ff99f49e\"},{\"content\":{\"connectorIds\":[\"Out1\",\"Out2\"],\"side\":\"TOP\"},\"type\":\"ConnectorPlacement.EquallySpacedRectSide\",\"uuid\":\"e62b0121-10a9-4e1e-945c-5e32104486a2\"}]},\"type\":\"ConnectorPlacement.EquallySpacedConnector\",\"uuid\":\"b7a6c70d-1829-427f-bdc0-db8f4193df4b\"}],\"packageUris\":[\"http://schema.mathworks.com/mf0/Connector/R2020b\"],\"version\":\"1.0\"}"
  mes9 : Subsystem
      settings: PortSchema="{\"entries\":[{\"content\":{\"sides\":[{\"content\":{\"connectorIds\":[\"LConn1\",\"LConn2\"]},\"type\":\"ConnectorPlacement.EquallySpacedRectSide\",\"uuid\":\"063d70f7-53e6-4b16-b677-e8cc0b373f72\"},{\"content\":{\"connectorIds\":[\"RConn1\",\"RConn2\"],\"side\":\"RIGHT\"},\"type\":\"ConnectorPlacement.EquallySpacedRectSide\",\"uuid\":\"e5801cd5-69d1-49e6-883b-eb22ff99f49e\"},{\"content\":{\"connectorIds\":[\"Out1\",\"Out2\"],\"side\":\"TOP\"},\"type\":\"ConnectorPlacement.EquallySpacedRectSide\",\"uuid\":\"e62b0121-10a9-4e1e-945c-5e32104486a2\"},{\"content\":{\"connectorIds\":[],\"side\":\"BOTTOM\"},\"type\":\"ConnectorPlacement.EquallySpacedRectSide\",\"uuid\":\"f5bc945b-430d-42e9-961b-d8bdce684df6\"}]},\"type\":\"ConnectorPlacement.EquallySpacedConnector\",\"uuid\":\"b7a6c70d-1829-427f-bdc0-db8f4193df4b\"}],\"packageUris\":[\"http://schema.mathworks.com/mf0/Connector/R2020b\"],\"version\":\"1.0\"}"
  powergui : spspowerguiLib/powergui  Priority=1  SimulationMode=Discrete  SampleTime=Ts_Power  frequency=60  Iterations=50  frequencyindice=0  Pbase=100e6  ErrMax=1e-4  UnitsV=kV  UnitsW=MW  buscounter=0  FunctionMessages=off  echomessages=off  EnableUseOfTLC=off  CurrentSourceSwitches=off  DisableSnubberDevices=off  DisableRonSwitches=off  DisableVfSwitches=off  DisplayEquations=off  AutomaticDiscreteSolvers=off  SolverType=Tustin/Backward Euler (TBE)  Interpol=off  ExternalGateDelay=off  methode=off  Ts=0  x0status=blocks  SPID=off  SwTol=0  HookPort=off  NonlinearTolerance=0  nMaxIteration=15  ContinueOnMaxIteration=off  RestoreLinks=warning  ResistiveCurrentMeasurement=off  Frange=[0:2:500]  Ylog=off  Xlog=on  ShowGrid=off  save=off  variable=ZData  structure=0  ZoomFFT=on  StartTime=0.0  cycles=1  DisplayStyle=1  fundamental=60  FreqAxis=off  MaxFrequency=1000  frequencyindicesteady=1  RmsSteady=1  display=off
  tag scope: P_pv=global, Vab_VSC=global, Vdc=global, m_PV=global, ratio_1=global, ratio_2=global, ratio_3=global
  wires:
  "Vdc "/1 -> [Vdc]
  [Vabc_B1] -> Inverter Control BN/1(Vabc_prim)
  [Iabc_B1] -> Inverter Control BN/2(Iabc_prim)
  [Vdc] -> Inverter Control BN/3(Vdc_mes)
  Inverter Control BN/1(Pulses) -> Product1/2
  Product1/1 -> FEC BN/1
  [I_PV] -> MPPT Controller/2(I_PV)
  [V_PV] -> MPPT Controller/1(V_PV)
  Pmean/1(P) -> [P_pv], "Ppv (kW) "/1, PV/3  "Pmean  (kW)"
  [m] -> VSC/2  "Mod. Index"
  Vdc 1/1 -> [Vab_VSC]
  [Vab_VSC] -> Vab_VSC/1
  [Ic_B1] -> Grid/2  "Ia (A)"
  [Vc_B1] -> Grid/1  "Va (V)"
  [P_B1_kW] -> P_trasf1/1, P trasformatore1(kW)/1  "P (kW)"
  Pmean/2(V) -> Vdc Boost/1, PV/4  "Vmean (V)"
  Subsystem2/2(VrVm) -> VSC/1  "Vref - Vmean"
  Subsystem2/1(Vm) -> Vdc Inverter/1
  [D] -> PV/5  "Duty Cycle"
  [Temp] -> PV/2  "Temp (deg. C)"
  [Ir] -> PV/1  "Ir (W/m^2)"
  [P_B0_kW] -> P_Inv1/1, P inverter1(kW)/1  "P (kW)"
  [Vdc] -> Inverter Control 1/3(Vdc_mes)
  [Iabc_B3] -> Inverter Control 1/2(Iabc_prim)
  [Vabc_B3] -> Inverter Control 1/1(Vabc_prim)
  [P_B2_kW] -> P inverter2(kW)/1, P_Inv2/1  "P (kW)"
  [P_B3_kW] -> P trasformatore2(kW)/1, P_trasf2/1  "P (kW)"
  [Vabc_B4] -> "Power to the load ramo 1 "/1
  [Iabc_B4] -> "Power to the load ramo 1 "/2
  "Power to the load ramo 1 "/1 -> "Load ramo 1 "/1
  "Load ramo 1 "/1 -> [Pload1], Mux1/1, P LOAD RAMO 1 (kW)/1, Saturation1/1
  [Vabc_B3] -> Power from the inverter 1/1
  [Iabc_B3] -> Power from the inverter 1/2
  Power from the inverter 1/1 -> P from inverter ramo 1/1
  P from inverter ramo 1/1 -> P INVERTER RAMO 1 (kW)/1, Mux1/2
  Mux1/1 -> P attiva ramo 1/1
  [Vabc_B5] -> Power from the grid/1
  [Iabc_B5] -> Power from the grid/2
  P from grid ramo 1/1 -> P GRID kW RAMO 1 (kW)/1, Mux1/3
  Power from the grid/1 -> P from grid ramo 1/1
  Inverter Control 1/1(Pulses) -> Product3/2
  Product3/1 -> FEC Unit.1/1
  Power to the load 1/1 -> P from grid1/1
  [Vabc_B1] -> Power to the load 1/1
  [Iabc_B1] -> Power to the load 1/2
  Power to the load 1/2 -> Terminator1/1
  [P_pv] -> Saturation/1
  Saturation/1 -> [Pinv]
  MATLAB Function/1(Pa) -> Demux/1
  [Pinv] -> MATLAB Function/2(Pinv)
  Demux/2 -> Divide4/1, Available Power Inverter 2/1
  Demux/1 -> Divide3/1, Available Power Inverter 1/1
  [Load_2] -> Mux/2
  [Load_3] -> Mux/3
  [Load_1] -> Mux/1
  Mux/1 -> MATLAB Function/1(Pload)
  Demux/3 -> Available Power Inverter 3/1, Divide5/1
  [Pinv] -> Divide3/2
  [Pinv] -> Divide4/2
  [Pinv] -> Divide5/2
  Divide4/1 -> [ratio_2]
  Divide5/1 -> [ratio_3]
  Divide3/1 -> [ratio_1]
  Saturation1/1 -> [Load_1]
  [Vdc] -> Inverter Control 2/3(Vdc_mes)
  mes1/2(v) -> [Vinv2]
  mes1/1(i) -> [Iinv2]
  mes3/1(i) -> [Iload2]
  mes4/1(i) -> [Igrid2]
  mes4/2(v) -> [Vgrid2]
  [Vinv2] -> Inverter Control 2/1(Vinv)
  [Iinv2] -> Inverter Control 2/2(Iinv)
  mes2/1(v) -> [Vsec2]
  mes3/2(v) -> [Vload2]
  Product4/1 -> FEC Unit. 2/1
  mes2/2(i) -> [Isec2]
  Inverter Control 2/1(Pulses) -> Product4/2
  Load ramo 2/1 -> Mux3/1, P LOAD RAMO 2 (kW)/1, Saturation2/1, [Pload2]
  Power from the inverter 2/2 -> Terminator4/1
  Mux3/1 -> P attiva ramo 2/1
  [Vload2] -> Power to the load ramo 2/1
  [Vsec2] -> Power from the inverter 2/1
  Saturation2/1 -> [Load_2]
  [Iload2] -> Power to the load ramo 2/2
  Power to the load ramo 2/1 -> Load ramo 2/1
  Power from the inverter 2/1 -> P from inverter ramo 2/1
  Power from the grid1/1 -> P from grid ramo 2/1
  [Igrid2] -> Power from the grid1/2
  [Isec2] -> Power from the inverter 2/2
  P from inverter ramo 2/1 -> P INVERTER RAMO 2 (kW)/1, Mux3/2
  [Vgrid2] -> Power from the grid1/1
  Power from the grid1/2 -> Terminator2/1
  Power to the load ramo 2/2 -> Terminator5/1
  [Iinv3] -> Inverter Control 3/2(Iinv)
  Inverter Control 3/1(g) -> Product5/2
  mes5/2(v) -> [Vinv3]
  [Vinv3] -> Inverter Control 3/1(Vinv)
  Product5/1 -> FEC Unit. 3/1
  mes6/2(i) -> [Isec3]
  mes9/1(v) -> [Vgrid3]
  mes9/2(i) -> [Igrid3]
  mes7/1(i) -> [Iload3]
  mes7/2(v) -> [Vload3]
  mes6/1(v) -> [Vsec3]
  mes5/1(i) -> [Iinv3]
  [Vdc] -> Inverter Control 3/3(Vdc_mes)
  Deblock Converters/1 -> Product1/1, Product5/1, Product4/1, Product3/1, Product2/2
  P from grid ramo 3/1 -> P GRID RAMO 3 (kW)/1, Mux4/3
  [Vsec3] -> Power from the inverter 3/1
  Power from the inverter 3/2 -> Terminator6/1
  P from inverter ramo 3/1 -> Mux4/2, P INVERTER RAMO 3 (kW)/1
  [Iload3] -> Power to the load ramo 3/2
  Power to the load ramo 3/1 -> Load ramo 3/1
  Power from the grid2/2 -> Terminator3/1
  Load ramo 3/1 -> P LOAD RAMO 3 (kW)/1, Saturation3/1, Mux4/1, [Pload3]
  Power to the load ramo 3/2 -> Terminator7/1
  Mux4/1 -> P attiva ramo 3/1
  [Igrid3] -> Power from the grid2/2
  Saturation3/1 -> [Load_3]
  [Vload3] -> Power to the load ramo 3/1
  [Isec3] -> Power from the inverter 3/2
  Power from the grid2/1 -> P from grid ramo 3/1
  Power from the inverter 3/1 -> P from inverter ramo 3/1
  [Vgrid3] -> Power from the grid2/1
  [P_pv] -> Balance Power System/1
  P from grid1/1 -> Potenza Attiva/1, P from grid2/1
  [Pload1] -> Balance Power System/2
  [Pload2] -> Balance Power System/3
  [Pload3] -> Balance Power System/4
  P from grid ramo 2/1 -> P GRID RAMO 2 (kW)/1, Mux3/3
  [Pbn] -> Balance Power System/5
  P from grid2/1 -> [Pbn]
  "Power to the load ramo 1 "/2 -> Terminator8/1
  Power from the inverter 1/2 -> Terminator9/1
  Power from the grid/2 -> Terminator10/1
  Product2/1 -> Subsystem/1(g)
  MPPT Controller/1(Pulses) -> Product2/1
  Subsystem3/1(m) -> [m_PV]
  connections:
  L_ba/RConn1 -- B0/LConn1 -- C_ba/LConn1
  L_ba/RConn2 -- B0/LConn2 -- C_ba/LConn2
  L_ba/RConn3 -- B0/LConn3 -- C_ba/LConn3
  C2/LConn1 -- FEC BN/RConn2 -- C1/RConn1
  B1/RConn3 -- " Load SC"/LConn3 -- B5/LConn3 -- mes4/RConn1 -- 600V Utlity Grid/LConn3
  Ground/LConn1 -- Vdc 1/LConn2
  FEC BN/LConn1 -- Vdc 1/LConn1 -- L_ba/LConn1
  FEC BN/LConn2 -- L_ba/LConn2
  FEC BN/LConn3 -- L_ba/LConn3
  TR_bn (30kVA)/RConn1 -- B0/RConn1
  TR_bn (30kVA)/RConn2 -- B0/RConn2
  TR_bn (30kVA)/RConn3 -- B0/RConn3
  TR_bn (30kVA)/LConn1 -- B1/LConn1
  TR_bn (30kVA)/LConn2 -- B1/LConn2
  TR_bn (30kVA)/LConn3 -- B1/LConn3
  C5/LConn1 -- C4/RConn1 -- FEC Unit.1/RConn2
  B4/LConn2 -- B3/RConn2 -- B5/RConn2
  B4/LConn1 -- B5/RConn1 -- B3/RConn1
  B4/LConn3 -- B5/RConn3 -- B3/RConn3
  "TR_10 kVA "/LConn3 -- B3/LConn3
  "TR_10 kVA "/LConn2 -- B3/LConn2
  "TR_10 kVA "/LConn1 -- B3/LConn1
  "TR_10 kVA "/RConn3 -- B2/RConn3
  "TR_10 kVA "/RConn2 -- B2/RConn2
  "TR_10 kVA "/RConn1 -- B2/RConn1
  L_ba1/LConn1 -- FEC Unit.1/LConn1
  C8/RConn1 -- FEC Unit. 2/RConn2 -- Subsystem/RConn2 -- "Vdc "/LConn2 -- FEC Unit. 3/RConn2 -- C9/RConn1 -- C5/RConn1 -- FEC Unit.1/RConn3 -- C2/RConn1 -- FEC BN/RConn3
  B1/RConn1 -- " Load SC"/LConn1 -- B5/LConn1 -- mes9/RConn1 -- 600V Utlity Grid/LConn1
  B1/RConn2 -- " Load SC"/LConn2 -- B5/LConn2 -- 600V Utlity Grid/LConn2
  " Load1"/LConn1 -- B4/RConn1
  " Load1"/LConn2 -- B4/RConn2
  " Load1"/LConn3 -- B4/RConn3
  L_ba1/LConn2 -- FEC Unit.1/LConn2
  L_ba1/LConn3 -- FEC Unit.1/LConn3
  L_ba1/RConn1 -- C_ba1/LConn3 -- B2/LConn1
  L_ba1/RConn2 -- C_ba1/LConn2 -- B2/LConn2
  L_ba1/RConn3 -- C_ba1/LConn1 -- B2/LConn3
  C6/RConn1 -- RL1/RConn1 -- mes1/LConn1
  mes2/RConn1 -- mes4/LConn1 -- mes3/LConn1
  TR_6kVA/LConn2 -- mes2/LConn1
  TR_6kVA/RConn2 -- mes1/RConn1
  Load 2/LConn1 -- mes3/RConn2
  FEC Unit. 2/LConn1 -- RL1/LConn1
  FEC Unit. 2/LConn2 -- C6/LConn1 -- mes1/LConn2
  mes5/LConn1 -- RL2/RConn1 -- C7/RConn1
  mes6/RConn1 -- mes9/LConn1 -- mes7/LConn2
  TR_3kVA/RConn1 -- mes5/RConn2
  TR_3kVA/LConn2 -- mes6/LConn1
  mes7/RConn2 -- " Load 3"/LConn1
  TR_3kVA/RConn2 -- mes5/RConn1
  mes5/LConn2 -- FEC Unit. 3/LConn2 -- C7/LConn1
  TR_6kVA/RConn1 -- mes1/RConn2
  TR_6kVA/LConn1 -- mes2/LConn2
  mes2/RConn2 -- mes3/LConn2 -- mes4/LConn2
  Load 2/RConn1 -- mes3/RConn1
  mes6/LConn2 -- TR_3kVA/LConn1
  " Load 3"/RConn1 -- mes7/RConn1
  mes7/LConn1 -- mes9/LConn2 -- mes6/RConn2
  FEC Unit. 2/RConn1 -- FEC BN/RConn1 -- C1/LConn1 -- FEC Unit.1/RConn1 -- C4/LConn1 -- C9/LConn1 -- FEC Unit. 3/RConn1 -- Subsystem/RConn1 -- "Vdc "/LConn1 -- C8/LConn1
  mes9/RConn2 -- mes4/RConn2 -- 600V Utlity Grid/RConn1
  FEC Unit. 3/LConn1 -- RL2/LConn1
  Subsystem3/RConn1 -- Subsystem/LConn1
  Subsystem3/RConn2 -- Subsystem/LConn2

== system PSMPraga/600V Utlity Grid ==
  400V 7MVA : spsThreePhaseSourceLib/Three-Phase Source  InternalConnection=Yn  VoltagePhases=off  Voltage=400  PhaseAngle=0  Voltage_phases=[25e3 25e3 25e3]/sqrt(3)  PhaseAngles_phases=[0 -120 +120]  Frequency=50  NonIdealSource=on  SpecifyImpedance=on  Resistance=0.8929  Inductance=16.58e-3  ShortCircuitLevel=7e6  BaseVoltage=400  XRratio=7  BusType=swing  Pref=0  Qref=0  Prefabc=[10e3, 10e3, 10e3]  Qrefabc=[0, 0, 0]  Qmin=-inf  Qmax=inf
  A : PMIOPort  Side=Left
  B : PMIOPort  Port=2  Side=Left
  C : PMIOPort  Port=3  Side=Left
  N : PMIOPort  Port=4  Side=Right
  connections:
  A/RConn1 -- 400V 7MVA/RConn1
  C/RConn1 -- 400V 7MVA/RConn3
  B/RConn1 -- 400V 7MVA/RConn2
  N/RConn1 -- 400V 7MVA/LConn1

== system PSMPraga/Inverter Control 1 ==
  note: VSC Main Controller
  Vabc_prim : Inport  PortDimensions=3
  Iabc_prim : Inport  Port=2  PortDimensions=3
  Vdc_mes : Inport  Port=3  PortDimensions=1
  Current Regulator : Subsystem
  Iq_ref : Constant  Value=0
  Mux : Mux  Inputs=2
  PLL & Measurements : Subsystem
  PWM Generator (3-Level) : spsPWMGenerator3LevelLib/PWM Generator (3-Level)  ModulatorType=Three-phase bridge (12 pulses)  ModulatorMode=Unsynchronized  nF=27  Fc=33*50  ModulatingSignals=off  m=0.8  Freq=60  Phase=0  Ts=Ts_Power
      settings: SourceProductBaseCode=PS
  Product : Product
  Saturation : Saturate  UpperLimit=1  LowerLimit=0
  Uabc_ref Generation max (m) = 1 : Subsystem
  Unit Delay : UnitDelay  SampleTime=Ts_Control  HasFrameUpgradeWarning=on
  VDC Regulator : Subsystem
  Vdc_ref1 : Constant  Value=Vdc_ref
  Pulses : Outport  VectorParamsAs1DForOutWhenUnconnected=off
  wires:
  Vdc_ref1/1 -> VDC Regulator/2(Vdc_ref)
  Uabc_ref Generation max (m) = 1/1(Uabc_ref) -> Unit Delay/1
  PWM Generator (3-Level)/1 -> Pulses/1
  Unit Delay/1 -> PWM Generator (3-Level)/1
  Iabc_prim/1 -> PLL & Measurements/2(Iabc_prim)
  Vabc_prim/1 -> PLL & Measurements/1(Vabc_prim)
  Vdc_mes/1 -> VDC Regulator/1(Vdc_mes)
  PLL & Measurements/2(VdVq_prim) -> Current Regulator/1(VdVq_mes)
  PLL & Measurements/3(IdIq_prim) -> Current Regulator/2(IdIq_mes)
  Mux/1 -> Current Regulator/3(IdIq_ref)
  Iq_ref/1 -> Mux/2
  Current Regulator/1(VdVq_conv) -> Uabc_ref Generation max (m) = 1/2(VdVq_conv)
  PLL & Measurements/1(wt) -> Uabc_ref Generation max (m) = 1/1(wt)
  [ratio_1] -> Saturation/1
  Product/1 -> Mux/1
  VDC Regulator/1(Id_ref) -> Product/1
  Saturation/1 -> Product/2

== system PSMPraga/Inverter Control 2 ==
  Vinv : Inport  PortDimensions=1
  Iinv : Inport  Port=2  PortDimensions=1
  Vdc_mes : Inport  Port=3  PortDimensions=1
  Current Regulator : Subsystem
  Iq_ref : Constant  Value=0
  Mux : Mux  Inputs=2
  PLL & Measurements : Subsystem
  PWM_Generator : spsPWMGenerator2LevelLib/PWM Generator (2-Level)  ModulatorType=Single-phase full-bridge - Bipolar modulation (4 pulses)  ModulatorMode=Unsynchronized  Fc=Fc  Pc=90  nF=27  MinMax="[ -1  1 ]"  SamplingTechnique=Natural  ModulatingSignals=off  m=0.8  Freq=60  Phase=0  Ts=Ts_Power  ShowCarrierOutport=off
      settings: AttributesFormatString=%<ModulatorType>
  Product : Product
  Saturation : Saturate  UpperLimit=1  LowerLimit=0
  "U_ref Generation " : Subsystem
  Unit Delay : UnitDelay  SampleTime=Ts_Control  HasFrameUpgradeWarning=on
  VDC Regulator : Subsystem
  Vnom_dc1 : Constant  Value=Vdc_ref
  Pulses : Outport  VectorParamsAs1DForOutWhenUnconnected=off
  wires:
  Iq_ref/1 -> Mux/2
  Vinv/1 -> PLL & Measurements/1(V_prim)
  Iinv/1 -> PLL & Measurements/2(I_prim)
  Unit Delay/1 -> PWM_Generator/1
  Mux/1 -> Current Regulator/3(IdIq_ref)
  Current Regulator/1(VdVq_conv) -> "U_ref Generation "/2(VdVq_conv)
  "U_ref Generation "/1(Uref) -> Unit Delay/1
  PWM_Generator/1 -> Pulses/1
  [ratio_2] -> Saturation/1
  PLL & Measurements/1(wt) -> "U_ref Generation "/1(wt)
  Vdc_mes/1 -> VDC Regulator/2(Vdc_mes)
  Vnom_dc1/1 -> VDC Regulator/1(Vdc_ref)
  PLL & Measurements/2(VdVq) -> Current Regulator/1(VdVq)
  PLL & Measurements/3(IdIq) -> Current Regulator/2(IdIq)
  VDC Regulator/1(Id_ref) -> Product/1
  Saturation/1 -> Product/2
  Product/1 -> Mux/1

== system PSMPraga/Inverter Control 3 ==
  Vinv : Inport  PortDimensions=1
  Iinv : Inport  Port=2  PortDimensions=1
  Vdc_mes : Inport  Port=3  PortDimensions=1
  Current Regulator : Subsystem
  Iq_ref : Constant  Value=0
  Mux : Mux  Inputs=2
  PLL & Measurements : Subsystem
  PWM_Generator : spsPWMGenerator2LevelLib/PWM Generator (2-Level)  ModulatorType=Single-phase full-bridge - Bipolar modulation (4 pulses)  ModulatorMode=Unsynchronized  Fc=Fc  Pc=90  nF=27  MinMax="[ -1  1 ]"  SamplingTechnique=Natural  ModulatingSignals=off  m=0.8  Freq=60  Phase=0  Ts=Ts_Power  ShowCarrierOutport=off
      settings: AttributesFormatString=%<ModulatorType>
  Product : Product
  Saturation : Saturate  UpperLimit=1  LowerLimit=0
  "U_ref Generation " : Subsystem
  Unit Delay : UnitDelay  SampleTime=Ts_Control  HasFrameUpgradeWarning=on
  VDC Regulator : Subsystem
  Vnom_dc1 : Constant  Value=Vdc_ref
  g : Outport  VectorParamsAs1DForOutWhenUnconnected=off
  wires:
  Iq_ref/1 -> Mux/2
  Vinv/1 -> PLL & Measurements/1(V_prim)
  Iinv/1 -> PLL & Measurements/2(I_prim)
  Unit Delay/1 -> PWM_Generator/1
  Mux/1 -> Current Regulator/3(IdIq_ref)
  Current Regulator/1(VdVq_conv) -> "U_ref Generation "/2(VdVq_conv)
  "U_ref Generation "/1(Uref) -> Unit Delay/1
  PWM_Generator/1 -> g/1
  [ratio_3] -> Saturation/1
  PLL & Measurements/1(wt) -> "U_ref Generation "/1(wt)
  Vdc_mes/1 -> VDC Regulator/2(Vdc_mes)
  Vnom_dc1/1 -> VDC Regulator/1(Vdc_ref)
  PLL & Measurements/2(VdVq) -> Current Regulator/1(VdVq)
  PLL & Measurements/3(IdIq) -> Current Regulator/2(IdIq)
  VDC Regulator/1(Id_ref) -> Product/1
  Saturation/1 -> Product/2
  Product/1 -> Mux/1
